simulink model "SimpleControlModel_NoAeroForces"  (R2019a)
settings: Solver=VariableStepAuto  StartTime=0.0  StopTime=10  RelTol=1e-3
InitFcn:
  | Inertia = [0.14 0 0;0 0.14 0;0 0 2e-4];
  | omega = [0;0;0];
  | wbw = 3;
  | 
  | I = sym('I', [3 3]);
  |     I = [I(1) 0 0;0 I(2,2) 0; 0 0 I(3,3)];
  |     InverseI = sym('InverseI', [3 3]);
  |     g = sym('q', [3 1], 'real');
  |     w = sym('w', [3 1], 'real');
  |     Mb = sym('Mb', [3 1]);
  | 
  |     A = jacobian([I \ (Mb - cross(w,I*w)); 0.5 * w], [w; g]);
  |     B = jacobian([I \ (Mb - cross(w,I*w)); 0.5 * w], Mb);
  |     C = eye(6);
  |     D = zeros([6 3]);
  | 
  |     A = subs(A, I, Inertia);
  |     A = subs(A, InverseI, inv(Inertia));
  | 
  |     B = subs(B, I, Inertia);
  |     B = subs(B, InverseI, inv(Inertia));
  | 
  |     A = subs(A, w, omega);
  |     B = subs(B, w, omega);
  | 
  |     ASimulink = double(A);
  |     BSimulink = double(B);
  |     CSimulink = double(C);
  |     DSimulink = double(D);
  | 
  | 
  |     KSimulink = lqr(nocontrol, diag([1,1,0,25,25,eps]), 0.1)
  | KSimulink(abs(KSimulink)<1e-5)=0
values from neighbouring files (symbols this model uses):
  Ai2 = double(jacobian([Mb/ Ixx; 0.5 * w; g], [w; g; gi]))    [StateSpaceController.m]
  Bi2 = double(jacobian([Mb/ Ixx; 0.5 * w; g], Mb))    [StateSpaceController.m]
  Ci2 = eye(size(Ai2,1))    [StateSpaceController.m]
  Ki2 = lqr(Ai2, Bi2, Q, R)    [StateSpaceController.m]
  nocontrol = ss(A, B, C, D)    [StateSpaceController.m]
undefined symbols (not defined in the file or in its folder): KISimulink
libraries: simulink x6, sharedutil x5, aerolibutil x1, aerolibbdyn x1
settings Model: Creator=rag  LastModifiedBy=rag

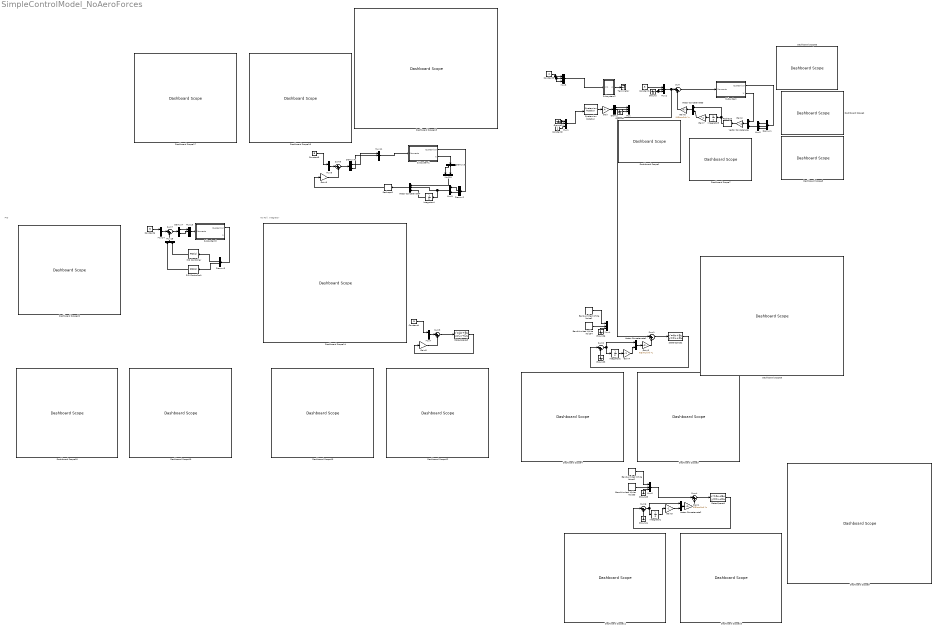
== system SimpleControlModel_NoAeroForces ==
  note: No Roll, Integrator
  note: PID
  Band-Limited White Noise1 : simulink/Sources/Band-Limited White Noise  Cov=[0.005]  Ts=0.5  seed=[23341]
  Band-Limited White Noise2 : simulink/Sources/Band-Limited White Noise  Cov=[0.005]  Ts=0.5  seed=[23341]
  Band-Limited White Noise3 : simulink/Sources/Band-Limited White Noise  Cov=[0.01]  Ts=1.2  seed=[19525]
  Band-Limited White Noise4 : simulink/Sources/Band-Limited White Noise  Cov=[0.01]  Ts=1.2  seed=[19525]
  Constant{1,4..6} (4 alike) : Constant  Value=.5
  Constant2 : Constant
  Constant3 : Constant  Value=.1
  Dashboard Scope{1..20} (20 alike) : DashboardScope
  Demux : Demux  Outputs=3
  Demux1 : Demux
  Demux2 : Demux
  Demux3 : Demux  Outputs=3
  Demux4 : Demux  Outputs=2
  Demux5 : Demux
  Demux7 : Demux  Outputs=2
  Gain : Gain  Gain=.4
  Gain1 : Gain  Gain=KISimulink  Multiplication=Matrix(K*u)
  Gain{2,4..5,7} (4 alike) : Gain  Gain=-1
  Gain3 : Gain  Gain=KISimulink  Multiplication=Matrix(K*u)
  Gain6 : Gain  Gain=KISimulink  Multiplication=Matrix(K*u)
  Gain8 : Gain  Gain=-Ki2  Multiplication=Matrix(K*u)
  Gain9 : Gain  Gain=-Ki2  Multiplication=Matrix(K*u)
  Ground{,1..6} (7 alike) : Ground
  Integrator{1..4} (4 alike) : Integrator
  Mux{,1..6,11,13} (9 alike) : Mux  Inputs=3
  Mux{7..10,14..15} (6 alike) : Mux  Inputs=2
  PID Controller : simulink/Continuous/PID Controller  Controller=PID  Form=Parallel  TimeDomain=Continuous-time  SampleTime=-1  IntegratorMethod=Forward Euler  FilterMethod=Forward Euler  ControllerParametersSource=internal  P=1  I=1  D=0  UseFilter=on  N=100  TunerSelectOption=Transfer Function Based (PID Tuner App)  InitialConditionSource=internal  InitialConditionForIntegrator=0  InitialConditionForFilter=0  DifferentiatorICPrevScaledInput=0  ExternalReset=none  TrackingMode=off  Kt=1  LimitOutput=off  UpperSaturationLimit=inf  LowerSaturationLimit=-inf  LinearizeAsGain=on  AntiWindupMode=none  Kb=1  POutMin=[]  POutMax=[]  IOutMin=[]  IOutMax=[]  DOutMin=[]  DOutMax=[]  NOutMin=[]  NOutMax=[]  SumOutMin=[]  SumOutMax=[]  SaturationOutMin=[]  SaturationOutMax=[]  PParamMin=[]  PParamMax=[]  IParamMin=[]  IParamMax=[]  DParamMin=[]  DParamMax=[]  NParamMin=[]  NParamMax=[]  KbParamMin=[]  KbParamMax=[]  KtParamMin=[]  KtParamMax=[]  KbOutMin=[]  KbOutMax=[]  KtOutMin=[]  KtOutMax=[]  IntegratorOutMin=[]  IntegratorOutMax=[]  FilterOutMin=[]  FilterOutMax=[]  SumI1OutMin=[]  SumI1OutMax=[]  SumI2OutMin=[]  SumI2OutMax=[]  SumI3OutMin=[]  SumI3OutMax=[]  SumI4OutMin=[]  SumI4OutMax=[]  SumDOutMin=[]  SumDOutMax=[]  DifferentiatorOutMin=[]  DifferentiatorOutMax=[]  FilterDiffOutCoefMin=[]  FilterDiffOutCoefMax=[]  ReciprocalOutMin=[]  ReciprocalOutMax=[]  SumDenOutMin=[]  SumDenOutMax=[]  SumNumOutMin=[]  SumNumOutMax=[]  DivideOutMin=[]  DivideOutMax=[]  IntegratorContinuousStateAttributes=''  IntegratorStateMustResolveToSignalObject=off  IntegratorRTWStateStorageClass=Auto  FilterContinuousStateAttributes=''  FilterStateMustResolveToSignalObject=off  FilterRTWStateStorageClass=Auto  ParallelPVariant=InternalParameters  IdealPVariant=Disabled  IVariant=InternalParameters  DVariant=InternalParameters  IntegratorVariant=Continuous  SatVariant=Disabled  AWVariant=Passthrough  PCopyVariant=Disabled  TRVariant=Disabled  FdbkBlocksVariant=Forward  IdealPFdbkVariant=Disabled  SatFdbkVariant=Disabled  DerivativeFilterVariant=ContFilter  NVariant=InternalParameters  NCopyVariant=Disabled  FilterICVariant=InternalICsFilter  IntegratorICVariant=InternalICs  ExternalResetVariant=Disabled  TRSumVariant=Passthrough  SumFdbkVariant=Disabled  SumVariant=Sum_PID
  PID Controller1 : simulink/Continuous/PID Controller  Controller=PID  Form=Parallel  TimeDomain=Continuous-time  SampleTime=-1  IntegratorMethod=Forward Euler  FilterMethod=Forward Euler  ControllerParametersSource=internal  P=1  I=1  D=0  UseFilter=on  N=100  TunerSelectOption=Transfer Function Based (PID Tuner App)  InitialConditionSource=internal  InitialConditionForIntegrator=0  InitialConditionForFilter=0  DifferentiatorICPrevScaledInput=0  ExternalReset=none  TrackingMode=off  Kt=1  LimitOutput=off  UpperSaturationLimit=inf  LowerSaturationLimit=-inf  LinearizeAsGain=on  AntiWindupMode=none  Kb=1  POutMin=[]  POutMax=[]  IOutMin=[]  IOutMax=[]  DOutMin=[]  DOutMax=[]  NOutMin=[]  NOutMax=[]  SumOutMin=[]  SumOutMax=[]  SaturationOutMin=[]  SaturationOutMax=[]  PParamMin=[]  PParamMax=[]  IParamMin=[]  IParamMax=[]  DParamMin=[]  DParamMax=[]  NParamMin=[]  NParamMax=[]  KbParamMin=[]  KbParamMax=[]  KtParamMin=[]  KtParamMax=[]  KbOutMin=[]  KbOutMax=[]  KtOutMin=[]  KtOutMax=[]  IntegratorOutMin=[]  IntegratorOutMax=[]  FilterOutMin=[]  FilterOutMax=[]  SumI1OutMin=[]  SumI1OutMax=[]  SumI2OutMin=[]  SumI2OutMax=[]  SumI3OutMin=[]  SumI3OutMax=[]  SumI4OutMin=[]  SumI4OutMax=[]  SumDOutMin=[]  SumDOutMax=[]  DifferentiatorOutMin=[]  DifferentiatorOutMax=[]  FilterDiffOutCoefMin=[]  FilterDiffOutCoefMax=[]  ReciprocalOutMin=[]  ReciprocalOutMax=[]  SumDenOutMin=[]  SumDenOutMax=[]  SumNumOutMin=[]  SumNumOutMax=[]  DivideOutMin=[]  DivideOutMax=[]  IntegratorContinuousStateAttributes=''  IntegratorStateMustResolveToSignalObject=off  IntegratorRTWStateStorageClass=Auto  FilterContinuousStateAttributes=''  FilterStateMustResolveToSignalObject=off  FilterRTWStateStorageClass=Auto  ParallelPVariant=InternalParameters  IdealPVariant=Disabled  IVariant=InternalParameters  DVariant=InternalParameters  IntegratorVariant=Continuous  SatVariant=Disabled  AWVariant=Passthrough  PCopyVariant=Disabled  TRVariant=Disabled  FdbkBlocksVariant=Forward  IdealPFdbkVariant=Disabled  SatFdbkVariant=Disabled  DerivativeFilterVariant=ContFilter  NVariant=InternalParameters  NCopyVariant=Disabled  FilterICVariant=InternalICsFilter  IntegratorICVariant=InternalICs  ExternalResetVariant=Disabled  TRSumVariant=Passthrough  SumFdbkVariant=Disabled  SumVariant=Sum_PID
  Quaternion Rotation : aerolibutil/Quaternion Rotation
  Reshape : Reshape  OutputDimensionality=Column vector (2-D)
  Reshape1 : Reshape  OutputDimensionality=Column vector (2-D)
  State-Space1 : StateSpace  A=ASimulink  B=BSimulink  C=CSimulink  D=DSimulink  InitialCondition=0
  State-Space2 : StateSpace  A=ASimulink  B=BSimulink  C=CSimulink  D=DSimulink  InitialCondition=0
  State-Space3 : StateSpace  A=Ai2  B=Bi2  C=Ci2  D=zeros(6,2)  InitialCondition=0
  Subsystem : Subsystem
  Subsystem1 : Subsystem
  Subsystem2 : Subsystem
  Subsystem3 : Subsystem
  Sum{,1,3..5,7} (6 alike) : Sum  Inputs=|++
  Sum2 : Sum  Inputs=|-+
  Sum6 : Sum  Inputs=|-+
  Terminator : Terminator
  Vector Concatenate{,1..3} (4 alike) : Concatenate
  Vector Concatenate4 : Concatenate  NumInputs=3
  wires:
  Demux/1 -> Mux/1
  Demux/2 -> Mux/2
  Ground1/1 -> Mux/3
  Quaternion Rotation/1 -> Gain/1
  Gain/1 -> Demux/1
  Mux1/1 -> Quaternion Rotation/2
  Ground2/1 -> Mux1/2, Mux1/1
  Constant2/1 -> Mux1/3
  Subsystem/2(w) -> Vector Concatenate/1
  Constant1/1 -> Mux2/1
  Ground/1 -> Mux2/3, Mux2/2
  Subsystem2/1(w) -> Terminator/1
  Mux3/1 -> Subsystem2/1(In1)
  Constant3/1 -> Mux3/3, Mux3/2, Mux3/1
  Demux1/4 -> Mux5/3
  Demux1/3 -> Mux5/2
  Demux1/2 -> Mux5/1
  Gain2/1 -> Reshape/1
  Vector Concatenate/1 -> Gain2/1
  Mux5/1 -> Vector Concatenate/2
  Sum/1 -> Subsystem/1(Moments)
  Gain6/1 -> Sum/2
  Sum6/1 -> Vector Concatenate2/1, Integrator1/1
  Ground4/1 -> Sum6/2
  Band-Limited White Noise3/1 -> Mux6/2
  Band-Limited White Noise2/1 -> Mux6/1
  Sum4/1 -> State-Space1/1
  State-Space1/1 -> Sum6/1
  Ground5/1 -> Mux6/3
  Gain1/1 -> Sum4/2
  Mux6/1 -> Sum4/1
  Subsystem/1(Quaternion) -> Demux1/1
  Mux2/1 -> Sum1/1, Sum/1
  Integrator1/1 -> Gain5/1
  Vector Concatenate2/1 -> Gain1/1
  State-Space2/1 -> Sum2/1
  Vector Concatenate1/1 -> Gain3/1
  Integrator2/1 -> Gain4/1
  Sum1/1 -> State-Space2/1
  Ground6/1 -> Mux4/3
  Band-Limited White Noise1/1 -> Mux4/1
  Band-Limited White Noise4/1 -> Mux4/2
  Gain3/1 -> Sum1/2
  Sum2/1 -> Vector Concatenate1/1, Integrator2/1
  Ground3/1 -> Sum2/2
  Gain4/1 -> Vector Concatenate1/2
  Gain5/1 -> Vector Concatenate2/2
  Gain7/1 -> Vector Concatenate3/2
  Integrator3/1 -> Gain7/1
  Vector Concatenate3/1 -> Gain6/1
  Reshape/1 -> Vector Concatenate3/1, Integrator3/1
  Sum3/1 -> State-Space3/1
  Gain8/1 -> Sum3/2
  State-Space3/1 -> Gain8/1
  Constant4/1 -> Mux7/1
  Mux7/1 -> Sum3/1
  Reshape1/1 -> Gain9/1
  Gain9/1 -> Sum5/2
  Mux8/1 -> Sum5/1
  Constant5/1 -> Mux8/1
  Subsystem1/1(Quaternion) -> Demux2/1
  Vector Concatenate4/1 -> Reshape1/1
  Sum5/1 -> Demux4/1
  Demux2/2 -> Mux9/1
  Subsystem1/2(w) -> Demux3/1
  Mux9/1 -> Integrator4/1, Vector Concatenate4/2
  Demux2/3 -> Mux9/2
  Demux3/2 -> Mux10/2
  Demux3/1 -> Mux10/1
  Mux10/1 -> Vector Concatenate4/1
  Integrator4/1 -> Vector Concatenate4/3
  Demux4/2 -> Mux11/2
  Demux4/1 -> Mux11/1
  Mux11/1 -> Subsystem1/1(Moments)
  Constant6/1 -> Mux14/1
  Demux5/2 -> PID Controller/1
  Sum7/1 -> Demux7/1
  Mux14/1 -> Sum7/1
  Mux13/1 -> Subsystem3/1(Moments)
  Demux7/1 -> Mux13/1
  Mux15/1 -> Sum7/2
  Demux7/2 -> Mux13/2
  Subsystem3/1(Quaternion) -> Demux5/1
  Demux5/3 -> PID Controller1/1
  PID Controller1/1 -> Mux15/1
  PID Controller/1 -> Mux15/2

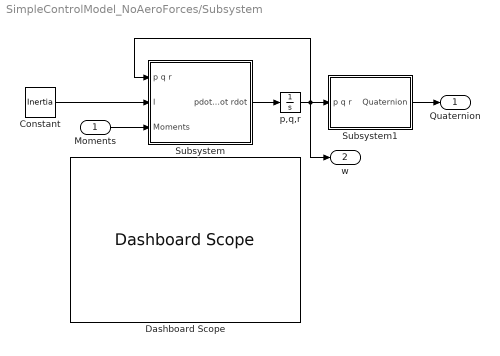
== system SimpleControlModel_NoAeroForces/Subsystem ==
  Moments : Inport  Unit=N*m  PortDimensions=3
  Constant : Constant  Value=Inertia
  Dashboard Scope : DashboardScope
  Subsystem : Subsystem
  Subsystem1 : Subsystem
  p,q,r : Integrator
  Quaternion : Outport
  w : Outport  Port=2
  wires:
  p,q,r/1 -> w/1, Subsystem1/1(p q r), Subsystem/1(p q r)
  Subsystem1/1(Quaternion) -> Quaternion/1
  Moments/1 -> Subsystem/3(Moments)
  Constant/1 -> Subsystem/2(I)
  Subsystem/1(pdot qdot rdot) -> p,q,r/1

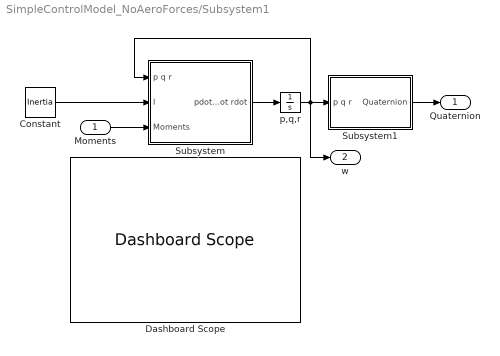
== system SimpleControlModel_NoAeroForces/Subsystem1 ==
  Moments : Inport  Unit=N*m  PortDimensions=3
  Constant : Constant  Value=Inertia
  Dashboard Scope : DashboardScope
  Subsystem : Subsystem
  Subsystem1 : Subsystem
  p,q,r : Integrator
  Quaternion : Outport
  w : Outport  Port=2
  wires:
  p,q,r/1 -> w/1, Subsystem1/1(p q r), Subsystem/1(p q r)
  Subsystem1/1(Quaternion) -> Quaternion/1
  Moments/1 -> Subsystem/3(Moments)
  Constant/1 -> Subsystem/2(I)
  Subsystem/1(pdot qdot rdot) -> p,q,r/1

== system SimpleControlModel_NoAeroForces/Subsystem2 ==
  In1 : Inport
  I : Subsystem
  Subsystem1 : Subsystem
  p,q,r : Integrator
  w : Outport
  wires:
  I/1(Out1) -> Subsystem1/2(I)
  Subsystem1/1(pdot qdot rdot) -> p,q,r/1
  In1/1 -> Subsystem1/3(Moments)
  p,q,r/1 -> w/1, Subsystem1/1(p q r)

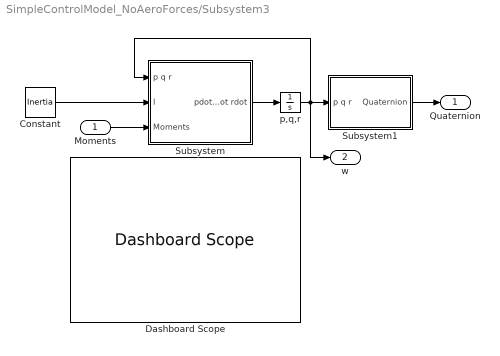
== system SimpleControlModel_NoAeroForces/Subsystem3 ==
  Moments : Inport  Unit=N*m  PortDimensions=3
  Constant : Constant  Value=Inertia
  Dashboard Scope : DashboardScope
  Subsystem : Subsystem
  Subsystem1 : Subsystem
  p,q,r : Integrator
  Quaternion : Outport
  w : Outport  Port=2
  wires:
  p,q,r/1 -> w/1, Subsystem1/1(p q r), Subsystem/1(p q r)
  Subsystem1/1(Quaternion) -> Quaternion/1
  Moments/1 -> Subsystem/3(Moments)
  Constant/1 -> Subsystem/2(I)
  Subsystem/1(pdot qdot rdot) -> p,q,r/1

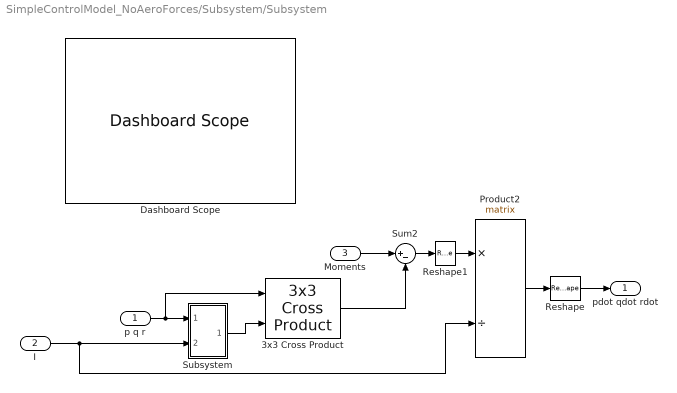
== system SimpleControlModel_NoAeroForces/Subsystem/Subsystem ==
  p q r : Inport
  I : Inport  Port=2
  Moments : Inport  Port=3
  3x3 Cross Product : sharedutil/3x3 Cross Product  aMode=aMode
      settings: SourceProductBaseCode=AE
  Dashboard Scope : DashboardScope
  Product2 : Product  Inputs=*/  Multiplication=Matrix(*)  SaturateOnIntegerOverflow=on  OutDataTypeStr=Inherit: Same as first input
  Reshape : Reshape
  Reshape1 : Reshape  OutputDimensionality=Row vector (2-D)
  Subsystem : Subsystem
  Sum2 : Sum  Inputs=|+-  SaturateOnIntegerOverflow=on
  pdot qdot rdot : Outport
  wires:
  Moments/1 -> Sum2/1
  Reshape1/1 -> Product2/1
  I/1 -> Subsystem/2(Inertia), Product2/2
  Sum2/1 -> Reshape1/1
  p q r/1 -> Subsystem/1(p q r1), 3x3 Cross Product/1
  Product2/1 -> Reshape/1
  Reshape/1 -> pdot qdot rdot/1
  Subsystem/1(I * w) -> 3x3 Cross Product/2
  3x3 Cross Product/1 -> Sum2/2

== system SimpleControlModel_NoAeroForces/Subsystem/Subsystem1 ==
  p q r : Inport
  Quaternion Normalize : sharedutil/Quaternion Normalize  aMode=aMode
      settings: SourceProductName=Aerospace Blockset  SourceProductBaseCode=AE
  Subsystem : Subsystem
  q0 q1 q2 q3 : Integrator  InitialCondition=[1, 0, 0, 0]
  Quaternion : Outport
  wires:
  Subsystem/1(qdot1) -> q0 q1 q2 q3/1
  p q r/1 -> Subsystem/1(p q r1)
  q0 q1 q2 q3/1 -> Quaternion Normalize/1
  Quaternion Normalize/1 -> Subsystem/2(q0 q1 q2 q1), Quaternion/1

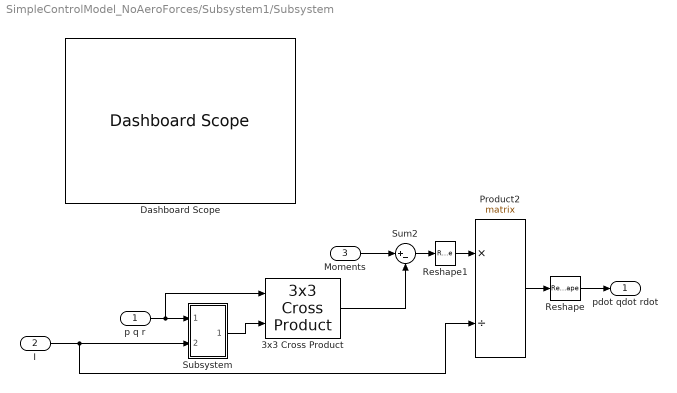
== system SimpleControlModel_NoAeroForces/Subsystem1/Subsystem ==
  p q r : Inport
  I : Inport  Port=2
  Moments : Inport  Port=3
  3x3 Cross Product : sharedutil/3x3 Cross Product  aMode=aMode
      settings: SourceProductBaseCode=AE
  Dashboard Scope : DashboardScope
  Product2 : Product  Inputs=*/  Multiplication=Matrix(*)  SaturateOnIntegerOverflow=on  OutDataTypeStr=Inherit: Same as first input
  Reshape : Reshape
  Reshape1 : Reshape  OutputDimensionality=Row vector (2-D)
  Subsystem : Subsystem
  Sum2 : Sum  Inputs=|+-  SaturateOnIntegerOverflow=on
  pdot qdot rdot : Outport
  wires:
  Moments/1 -> Sum2/1
  Reshape1/1 -> Product2/1
  I/1 -> Subsystem/2(Inertia), Product2/2
  Sum2/1 -> Reshape1/1
  p q r/1 -> Subsystem/1(p q r1), 3x3 Cross Product/1
  Product2/1 -> Reshape/1
  Reshape/1 -> pdot qdot rdot/1
  Subsystem/1(I * w) -> 3x3 Cross Product/2
  3x3 Cross Product/1 -> Sum2/2

== system SimpleControlModel_NoAeroForces/Subsystem1/Subsystem1 ==
  p q r : Inport
  Subsystem : Subsystem
  q0 q1 q2 q3 : Integrator  InitialCondition=[1, 0, 0, 0]
  Quaternion : Outport
  wires:
  Subsystem/1(qdot1) -> q0 q1 q2 q3/1
  p q r/1 -> Subsystem/1(p q r1)
  q0 q1 q2 q3/1 -> Subsystem/2(q0 q1 q2 q1), Quaternion/1

== system SimpleControlModel_NoAeroForces/Subsystem2/I ==
  Constant : Constant  Value=0.13141
  Constant1 : Constant  Value=2.47E-04
  Ground : Ground
  Symmetric Inertia Tensor : aerolibbdyn/Symmetric Inertia Tensor
      settings: SourceProductName=Aerospace Blockset  SourceProductBaseCode=AE
  Out1 : Outport
  wires:
  Ground/1 -> Symmetric Inertia Tensor/5, Symmetric Inertia Tensor/3, Symmetric Inertia Tensor/2
  Constant1/1 -> Symmetric Inertia Tensor/6
  Constant/1 -> Symmetric Inertia Tensor/1, Symmetric Inertia Tensor/4
  Symmetric Inertia Tensor/1 -> Out1/1

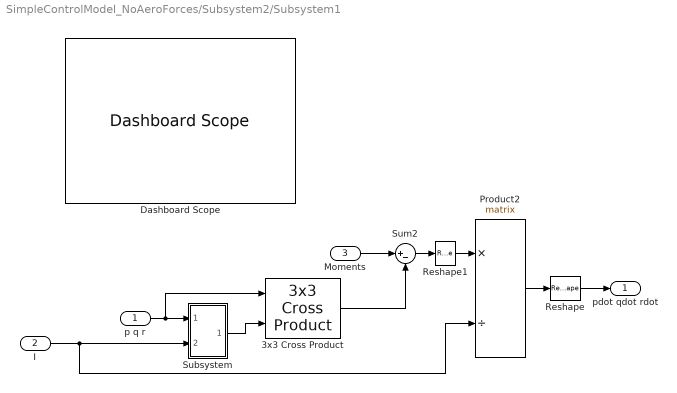
== system SimpleControlModel_NoAeroForces/Subsystem2/Subsystem1 ==
  p q r : Inport
  I : Inport  Port=2
  Moments : Inport  Port=3
  3x3 Cross Product : sharedutil/3x3 Cross Product  aMode=aMode
      settings: SourceProductBaseCode=AE
  Dashboard Scope : DashboardScope
  Product2 : Product  Inputs=*/  Multiplication=Matrix(*)  SaturateOnIntegerOverflow=on  OutDataTypeStr=Inherit: Same as first input
  Reshape : Reshape
  Reshape1 : Reshape  OutputDimensionality=Row vector (2-D)
  Subsystem : Subsystem
  Sum2 : Sum  Inputs=|+-  SaturateOnIntegerOverflow=on
  pdot qdot rdot : Outport
  wires:
  Moments/1 -> Sum2/1
  Reshape1/1 -> Product2/1
  I/1 -> Subsystem/2(Inertia), Product2/2
  Sum2/1 -> Reshape1/1
  p q r/1 -> Subsystem/1(p q r1), 3x3 Cross Product/1
  Product2/1 -> Reshape/1
  Reshape/1 -> pdot qdot rdot/1
  Subsystem/1(I * w) -> 3x3 Cross Product/2
  3x3 Cross Product/1 -> Sum2/2

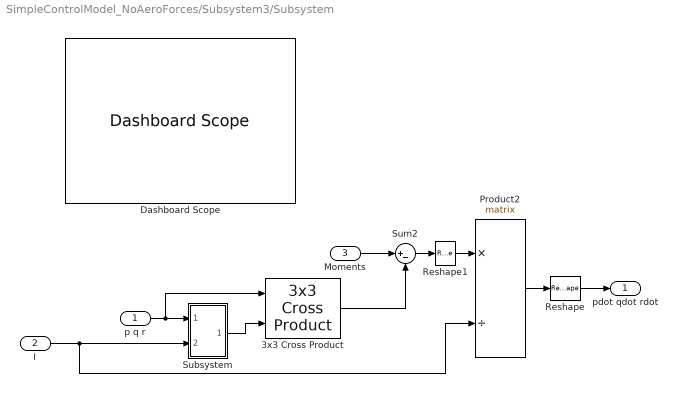
== system SimpleControlModel_NoAeroForces/Subsystem3/Subsystem ==
  p q r : Inport
  I : Inport  Port=2
  Moments : Inport  Port=3
  3x3 Cross Product : sharedutil/3x3 Cross Product  aMode=aMode
      settings: SourceProductBaseCode=AE
  Dashboard Scope : DashboardScope
  Product2 : Product  Inputs=*/  Multiplication=Matrix(*)  SaturateOnIntegerOverflow=on  OutDataTypeStr=Inherit: Same as first input
  Reshape : Reshape
  Reshape1 : Reshape  OutputDimensionality=Row vector (2-D)
  Subsystem : Subsystem
  Sum2 : Sum  Inputs=|+-  SaturateOnIntegerOverflow=on
  pdot qdot rdot : Outport
  wires:
  Moments/1 -> Sum2/1
  Reshape1/1 -> Product2/1
  I/1 -> Subsystem/2(Inertia), Product2/2
  Sum2/1 -> Reshape1/1
  p q r/1 -> Subsystem/1(p q r1), 3x3 Cross Product/1
  Product2/1 -> Reshape/1
  Reshape/1 -> pdot qdot rdot/1
  Subsystem/1(I * w) -> 3x3 Cross Product/2
  3x3 Cross Product/1 -> Sum2/2

== system SimpleControlModel_NoAeroForces/Subsystem3/Subsystem1 ==
  p q r : Inport
  Subsystem : Subsystem
  q0 q1 q2 q3 : Integrator  InitialCondition=[1, 0, 0, 0]
  Quaternion : Outport
  wires:
  Subsystem/1(qdot1) -> q0 q1 q2 q3/1
  p q r/1 -> Subsystem/1(p q r1)
  q0 q1 q2 q3/1 -> Subsystem/2(q0 q1 q2 q1), Quaternion/1

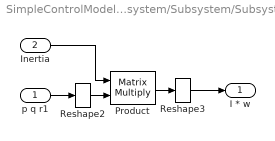
== system SimpleControlModel_NoAeroForces/Subsystem/Subsystem/Subsystem ==
  p q r1 : Inport
  Inertia : Inport  Port=2
  Product : Product  Multiplication=Matrix(*)  SaturateOnIntegerOverflow=on  InputSameDT=on  OutDataTypeStr=Inherit: Same as first input
  Reshape2 : Reshape  OutputDimensionality=Column vector (2-D)
  Reshape3 : Reshape
  I * w : Outport
  wires:
  p q r1/1 -> Reshape2/1
  Product/1 -> Reshape3/1
  Inertia/1 -> Product/1
  Reshape2/1 -> Product/2
  Reshape3/1 -> I * w/1

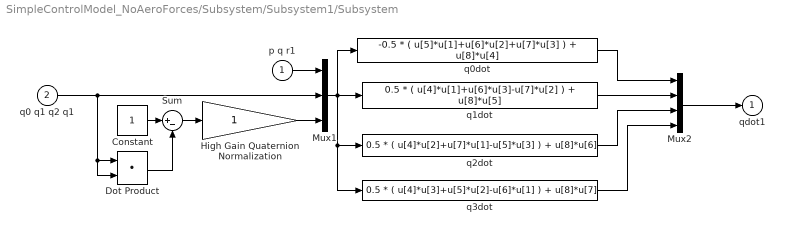
== system SimpleControlModel_NoAeroForces/Subsystem/Subsystem1/Subsystem ==
  p q r1 : Inport
  q0 q1 q2 q1 : Inport  Port=2  PortDimensions=4
  Constant : Constant
  Dot Product : DotProduct  OutDataTypeStr=Inherit: Inherit via internal rule
  High Gain Quaternion Normalization : Gain  SaturateOnIntegerOverflow=on  OutDataTypeStr=Inherit: Same as input  ParamDataTypeStr=Inherit: Same as input
  Mux1 : Mux  Inputs=[3 4 1]
  Mux2 : Mux
  Sum : Sum  Inputs=|+-  SaturateOnIntegerOverflow=on  InputSameDT=on  OutDataTypeStr=Inherit: Same as first input
  q0dot : Fcn  Expr=-0.5 * ( u[5]*u[1]+u[6]*u[2]+u[7]*u[3] ) + u[8]*u[4]
  q1dot : Fcn  Expr=0.5 * ( u[4]*u[1]+u[6]*u[3]-u[7]*u[2] ) + u[8]*u[5]
  q2dot : Fcn  Expr=0.5 * ( u[4]*u[2]+u[7]*u[1]-u[5]*u[3] ) + u[8]*u[6]
  q3dot : Fcn  Expr=0.5 * ( u[4]*u[3]+u[5]*u[2]-u[6]*u[1] ) + u[8]*u[7]
  qdot1 : Outport  InitialOutput=0
  wires:
  Mux2/1 -> qdot1/1
  Dot Product/1 -> Sum/2
  q3dot/1 -> Mux2/4
  High Gain Quaternion Normalization/1 -> Mux1/3
  Mux1/1 -> q2dot/1, q3dot/1, q0dot/1, q1dot/1
  q1dot/1 -> Mux2/2
  q2dot/1 -> Mux2/3
  Constant/1 -> Sum/1
  Sum/1 -> High Gain Quaternion Normalization/1
  p q r1/1 -> Mux1/1
  q0dot/1 -> Mux2/1
  q0 q1 q2 q1/1 -> Dot Product/1, Dot Product/2, Mux1/2

== system SimpleControlModel_NoAeroForces/Subsystem1/Subsystem/Subsystem ==
  p q r1 : Inport
  Inertia : Inport  Port=2
  Product : Product  Multiplication=Matrix(*)  SaturateOnIntegerOverflow=on  InputSameDT=on  OutDataTypeStr=Inherit: Same as first input
  Reshape2 : Reshape  OutputDimensionality=Column vector (2-D)
  Reshape3 : Reshape
  I * w : Outport
  wires:
  p q r1/1 -> Reshape2/1
  Product/1 -> Reshape3/1
  Inertia/1 -> Product/1
  Reshape2/1 -> Product/2
  Reshape3/1 -> I * w/1

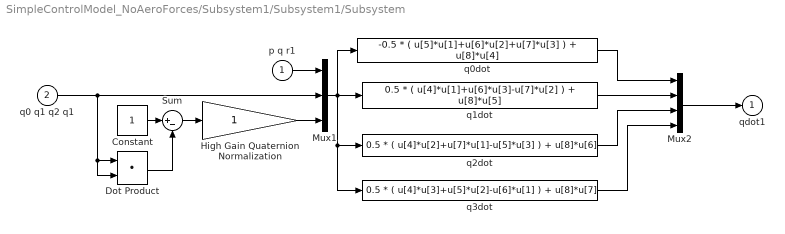
== system SimpleControlModel_NoAeroForces/Subsystem1/Subsystem1/Subsystem ==
  p q r1 : Inport
  q0 q1 q2 q1 : Inport  Port=2  PortDimensions=4
  Constant : Constant
  Dot Product : DotProduct  OutDataTypeStr=Inherit: Inherit via internal rule
  High Gain Quaternion Normalization : Gain  SaturateOnIntegerOverflow=on  OutDataTypeStr=Inherit: Same as input  ParamDataTypeStr=Inherit: Same as input
  Mux1 : Mux  Inputs=[3 4 1]
  Mux2 : Mux
  Sum : Sum  Inputs=|+-  SaturateOnIntegerOverflow=on  InputSameDT=on  OutDataTypeStr=Inherit: Same as first input
  q0dot : Fcn  Expr=-0.5 * ( u[5]*u[1]+u[6]*u[2]+u[7]*u[3] ) + u[8]*u[4]
  q1dot : Fcn  Expr=0.5 * ( u[4]*u[1]+u[6]*u[3]-u[7]*u[2] ) + u[8]*u[5]
  q2dot : Fcn  Expr=0.5 * ( u[4]*u[2]+u[7]*u[1]-u[5]*u[3] ) + u[8]*u[6]
  q3dot : Fcn  Expr=0.5 * ( u[4]*u[3]+u[5]*u[2]-u[6]*u[1] ) + u[8]*u[7]
  qdot1 : Outport  InitialOutput=0
  wires:
  Mux2/1 -> qdot1/1
  Dot Product/1 -> Sum/2
  q3dot/1 -> Mux2/4
  High Gain Quaternion Normalization/1 -> Mux1/3
  Mux1/1 -> q2dot/1, q3dot/1, q0dot/1, q1dot/1
  q1dot/1 -> Mux2/2
  q2dot/1 -> Mux2/3
  Constant/1 -> Sum/1
  Sum/1 -> High Gain Quaternion Normalization/1
  p q r1/1 -> Mux1/1
  q0dot/1 -> Mux2/1
  q0 q1 q2 q1/1 -> Dot Product/1, Dot Product/2, Mux1/2

== system SimpleControlModel_NoAeroForces/Subsystem2/Subsystem1/Subsystem ==
  p q r1 : Inport
  Inertia : Inport  Port=2
  Product : Product  Multiplication=Matrix(*)  SaturateOnIntegerOverflow=on  InputSameDT=on  OutDataTypeStr=Inherit: Same as first input
  Reshape2 : Reshape  OutputDimensionality=Column vector (2-D)
  Reshape3 : Reshape
  I * w : Outport
  wires:
  p q r1/1 -> Reshape2/1
  Product/1 -> Reshape3/1
  Inertia/1 -> Product/1
  Reshape2/1 -> Product/2
  Reshape3/1 -> I * w/1

== system SimpleControlModel_NoAeroForces/Subsystem3/Subsystem/Subsystem ==
  p q r1 : Inport
  Inertia : Inport  Port=2
  Product : Product  Multiplication=Matrix(*)  SaturateOnIntegerOverflow=on  InputSameDT=on  OutDataTypeStr=Inherit: Same as first input
  Reshape2 : Reshape  OutputDimensionality=Column vector (2-D)
  Reshape3 : Reshape
  I * w : Outport
  wires:
  p q r1/1 -> Reshape2/1
  Product/1 -> Reshape3/1
  Inertia/1 -> Product/1
  Reshape2/1 -> Product/2
  Reshape3/1 -> I * w/1

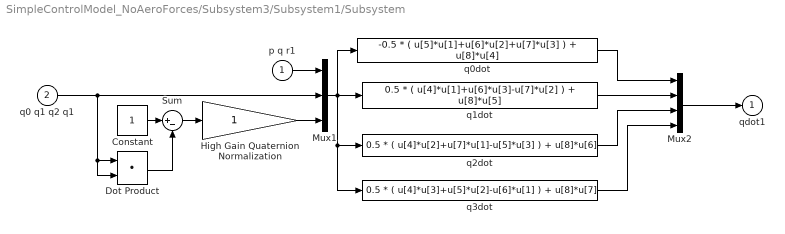
== system SimpleControlModel_NoAeroForces/Subsystem3/Subsystem1/Subsystem ==
  p q r1 : Inport
  q0 q1 q2 q1 : Inport  Port=2  PortDimensions=4
  Constant : Constant
  Dot Product : DotProduct  OutDataTypeStr=Inherit: Inherit via internal rule
  High Gain Quaternion Normalization : Gain  SaturateOnIntegerOverflow=on  OutDataTypeStr=Inherit: Same as input  ParamDataTypeStr=Inherit: Same as input
  Mux1 : Mux  Inputs=[3 4 1]
  Mux2 : Mux
  Sum : Sum  Inputs=|+-  SaturateOnIntegerOverflow=on  InputSameDT=on  OutDataTypeStr=Inherit: Same as first input
  q0dot : Fcn  Expr=-0.5 * ( u[5]*u[1]+u[6]*u[2]+u[7]*u[3] ) + u[8]*u[4]
  q1dot : Fcn  Expr=0.5 * ( u[4]*u[1]+u[6]*u[3]-u[7]*u[2] ) + u[8]*u[5]
  q2dot : Fcn  Expr=0.5 * ( u[4]*u[2]+u[7]*u[1]-u[5]*u[3] ) + u[8]*u[6]
  q3dot : Fcn  Expr=0.5 * ( u[4]*u[3]+u[5]*u[2]-u[6]*u[1] ) + u[8]*u[7]
  qdot1 : Outport  InitialOutput=0
  wires:
  Mux2/1 -> qdot1/1
  Dot Product/1 -> Sum/2
  q3dot/1 -> Mux2/4
  High Gain Quaternion Normalization/1 -> Mux1/3
  Mux1/1 -> q2dot/1, q3dot/1, q0dot/1, q1dot/1
  q1dot/1 -> Mux2/2
  q2dot/1 -> Mux2/3
  Constant/1 -> Sum/1
  Sum/1 -> High Gain Quaternion Normalization/1
  p q r1/1 -> Mux1/1
  q0dot/1 -> Mux2/1
  q0 q1 q2 q1/1 -> Dot Product/1, Dot Product/2, Mux1/2
